simulink model "Enabled_subsystem_test"  (R2022a)
settings: Solver=VariableStepAuto  StartTime=0.0  StopTime=10.0  RelTol=1e-3
settings Model: Creator=ADMIN  LastModifiedBy=ADMIN

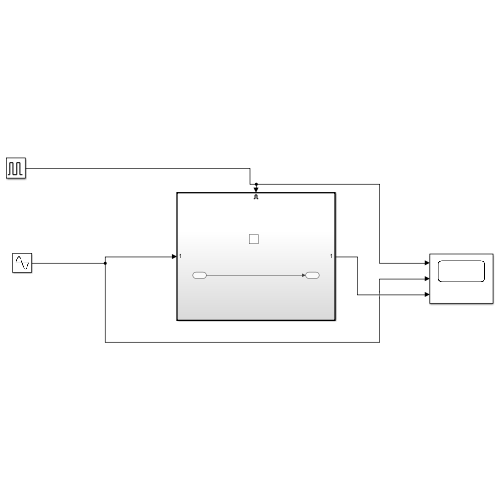
[thumbnail: Simulink's stored preview of the top-level diagram]
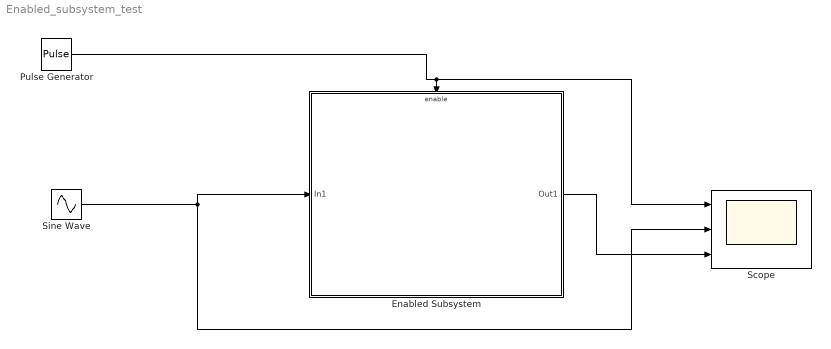
== system Enabled_subsystem_test ==
  Enabled Subsystem : Subsystem  TreatAsAtomicUnit=on
  Pulse Generator : DiscretePulseGenerator  PulseType=Time based  Period=1  PulseWidth=50
  Scope : Scope  NumInputPorts=3
  Sine Wave : Sin  Frequency=2*pi*1  SampleTime=0
  wires:
  Sine Wave/1 -> Scope/2, Enabled Subsystem/1(In1)
  Pulse Generator/1 -> Scope/1, Enabled Subsystem/Enable
  Enabled Subsystem/1(Out1) -> Scope/3

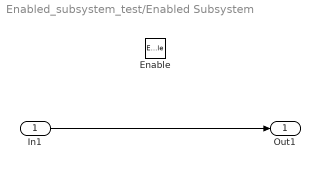
== system Enabled_subsystem_test/Enabled Subsystem ==
  In1 : Inport
  Enable : EnablePort
  Out1 : Outport
  wires:
  In1/1 -> Out1/1
